simulink model "Zadatak2"  (R2013b)
settings: Solver=ode45  StartTime=0.0  StopTime=0.1  RelTol=1e-3
settings Model: Creator=Korisnik  LastModifiedBy=Korisnik

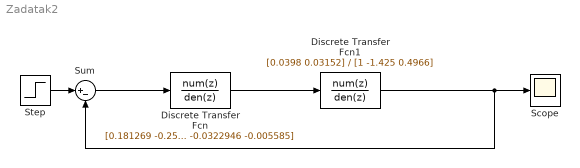
== system Zadatak2 ==
  Discrete Transfer Fcn : DiscreteTransferFcn  Numerator=[0.181269 -0.258127 0.089855]  Denominator=[0.039 -0.00112 -0.0322946 -0.005585]
  Discrete Transfer Fcn1 : DiscreteTransferFcn  Numerator=[0.0398 0.03152]  Denominator=[1 -1.425 0.4966]
  Scope : Scope
  Step : Step  SampleTime=0
  Sum : Sum  Inputs=|+-
  wires:
  Discrete Transfer Fcn1/1 -> Sum/2, Scope/1
  Step/1 -> Sum/1
  Sum/1 -> Discrete Transfer Fcn/1
  Discrete Transfer Fcn/1 -> Discrete Transfer Fcn1/1
